simulink model "pendulumTest"  (R2021a)
settings: Solver=VariableStepAuto  StartTime=0.0  StopTime=10.0  FixedStep=1/20000  RelTol=1e-3
InitFcn:
  | run('init.m');
values from neighbouring files (symbols this model uses):
  g = 9.81    [init.m]
  l = 0.5    [init.m]
  m = 1    [init.m]
  Q = 1e-5    (= 1e-05)    [init.m]
  R = 1e-3    (= 0.001)    [init.m]
  Ts = 1/2000    (= 0.0005)    [init.m]
undefined symbols (not defined in the file or in its folder): A, B, Discrete, H, Time, X, Y, Z
libraries: sm_lib x8, nesl_utility x3, simulink x2, ctrlSharedLib x1
settings Model: Creator=Max  LastModifiedBy=Max

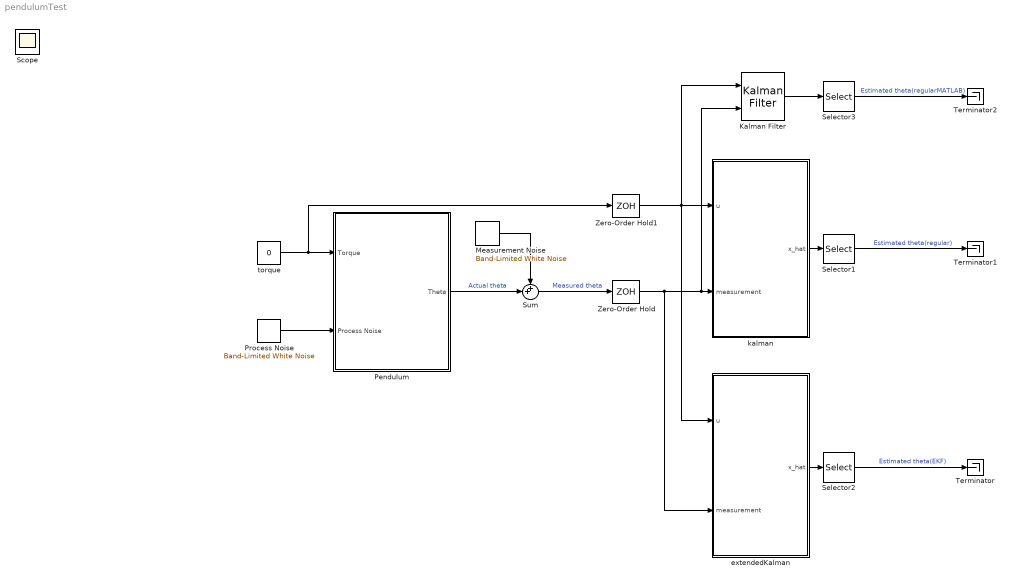
== system pendulumTest ==
  Kalman Filter : ctrlSharedLib/Kalman Filter  TimeDomain=Discrete-Time  UseCurrentEstimator=on  ModelSource=Individual A, B, C, D matrices  ModelSourceVariable=ss(0.95,1,1,0,1)  A=A  B=B  C=H  D=0  NumberOfStates=1  NumberOfInputs=1  NumberOfOutputs=1  InitialEstimateSource=Dialog  X0=0  P0=10  UseK=off  UseGH=off  NumberOfProcessNoiseInputs=1  G=1  TimeInvariantG=on  H=0  TimeInvariantH=on  Q=diag([0 Q])  TimeInvariantQ=on  R=R  TimeInvariantR=on  N=0  TimeInvariantN=on  AddInputPort=on  AddEnablePort=off  OutputEstimatedY=off  OutputP=off  Ts=Ts
  Measurement Noise : simulink/Sources/Band-Limited White Noise  Cov=R*Ts  Ts=Ts  seed=[12347]
  Pendulum : Subsystem  mask{theta_0=0.75*pi, theta_dot_0=0}
      mask prompts: theta_0 "Initial value of theta"; theta_dot_0 "Initial value of theta_dot"
      mask Display:
      | port_label('input',1,'T');
      | port_label('input',2,'w');
      | port_label('output',1,'\theta','interpreter','tex');
  Process Noise : simulink/Sources/Band-Limited White Noise  Cov=Q*Ts  Ts=Ts  seed=[23341]
  Selector1 : Selector  InputPortWidth=2  IndexOptions=Index vector (dialog)  Indices=1  OutputSizes=1
  Selector2 : Selector  InputPortWidth=2  IndexOptions=Index vector (dialog)  Indices=1  OutputSizes=1
  Selector3 : Selector  InputPortWidth=2  IndexOptions=Index vector (dialog)  Indices=1  OutputSizes=1
  Sum : Sum  Inputs=++|
  Terminator : Terminator
  Terminator1 : Terminator
  Terminator2 : Terminator
  Zero-Order Hold : ZeroOrderHold  SampleTime=Ts
  Zero-Order Hold1 : ZeroOrderHold  SampleTime=Ts
  extendedKalman : MATLAB Function  TreatAsAtomicUnit=on
  kalman : MATLAB Function  TreatAsAtomicUnit=on
  torque : Constant  Value=0
  Scope : Scope
  wires:
  kalman/1(x_hat) -> Selector1/1
  Pendulum/1(Theta) -> Sum/2  "Actual theta"
  Selector1/1 -> Terminator1/1  "Estimated theta(regular)"
  Sum/1 -> Zero-Order Hold/1  "Measured theta"
  Process Noise/1 -> Pendulum/2(Process Noise)
  Selector2/1 -> Terminator/1  "Estimated theta(EKF)"
  Measurement Noise/1 -> Sum/1
  torque/1 -> Pendulum/1(Torque), Zero-Order Hold1/1
  Zero-Order Hold/1 -> extendedKalman/2(measurement), Kalman Filter/2, kalman/2(measurement)
  Zero-Order Hold1/1 -> kalman/1(u), extendedKalman/1(u), Kalman Filter/1
  extendedKalman/1(x_hat) -> Selector2/1
  Kalman Filter/1 -> Selector3/1
  Selector3/1 -> Terminator2/1  "Estimated theta(regularMATLAB)"

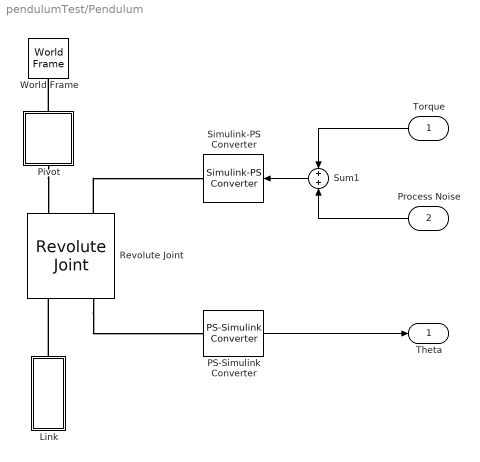
== system pendulumTest/Pendulum ==
  Torque : Inport
  Process Noise : Inport  Port=2
  Link : Subsystem  Tag=CustomStyle
  PS-Simulink Converter : nesl_utility/PS-Simulink Converter  PhysicalDomain=network_engine_domain  SubClassName=ps_output  LeftPortType=input  RightPortType=output  PseudoPeriodic=off  Frequencies=[]  Unit=1  AffineConversion=off
  Pivot : Subsystem  Tag=CustomStyle
  Revolute Joint : sm_lib/Joints/Revolute Joint  JointMode=Normal  SenseConstraintForce=off  SenseConstraintForceX=off  SenseConstraintForceY=off  SenseConstraintForceZ=off  SenseConstraintTorque=off  SenseConstraintTorqueX=off  SenseConstraintTorqueY=off  SenseConstraintTorqueZ=off  SenseTotalForce=off  SenseTotalForceX=off  SenseTotalForceY=off  SenseTotalForceZ=off  SenseTotalTorque=off  SenseTotalTorqueX=off  SenseTotalTorqueY=off  SenseTotalTorqueZ=off  CompositeWrenchDir=FollowerOnBase  CompositeWrenchFrame=BaseFrame  EquilibriumPosition=0  EquilibriumPositionUnits=rad  SpringStiffness=0  SpringStiffnessUnits=N*m/rad  DampingCoefficient=0  DampingCoefficientUnits=N*m/(rad/s)  TorqueActuationMode=InputTorque  MotionActuationMode=ComputedMotion  SensePosition=on  SenseVelocity=off  SenseAcceleration=off  SenseTorqueForce=off  SenseLowerLimitTorqueForce=off  SenseUpperLimitTorqueForce=off  LowerLimitSpecify=off  LowerLimitBound=-90  LowerLimitBoundUnits=deg  LowerLimitStiffness=1e4  LowerLimitStiffnessUnits=N*m/deg  LowerLimitDamping=10  LowerLimitDampingUnits=N*m/(deg/s)  LowerLimitTransitionRegionWidth=0.1  LowerLimitTransitionRegionWidthUnits=deg  UpperLimitSpecify=off  UpperLimitBound=90  UpperLimitBoundUnits=deg  UpperLimitStiffness=1e4  UpperLimitStiffnessUnits=N*m/deg  UpperLimitDamping=10  UpperLimitDampingUnits=N*m/(deg/s)  UpperLimitTransitionRegionWidth=0.1  UpperLimitTransitionRegionWidthUnits=deg  PositionTargetSpecify=on  PositionTargetPriority=High  PositionTargetValue=theta_0  PositionTargetValueUnits=rad  VelocityTargetSpecify=on  VelocityTargetPriority=High  VelocityTargetValue=theta_dot_0  VelocityTargetValueUnits=rad/s
  Simulink-PS Converter : nesl_utility/Simulink-PS Converter  PhysicalDomain=network_engine_domain  SubClassName=ps_input  LeftPortType=input  RightPortType=output  PseudoPeriodic=off  Frequencies=[]  NoiseDistribution=none  NoiseParameters=[]  Unit=1  AffineConversion=off  FilteringAndDerivatives=provide  SimscapeFilterOrder=1  InputFilterTimeConstant=0.001  UdotUserProvided=0
  Sum1 : Sum  Inputs=+|+
  World Frame : sm_lib/Frames and Transforms/World Frame
  Theta : Outport
  wires:
  Sum1/1 -> Simulink-PS Converter/1
  Torque/1 -> Sum1/1
  Process Noise/1 -> Sum1/2
  PS-Simulink Converter/1 -> Theta/1
  connections:
  Revolute Joint/LConn2 -- Simulink-PS Converter/RConn1
  Pivot/LConn1 -- World Frame/RConn1
  Pivot/RConn1 -- Revolute Joint/LConn1
  Link/RConn1 -- Revolute Joint/RConn1
  Revolute Joint/RConn2 -- PS-Simulink Converter/LConn1

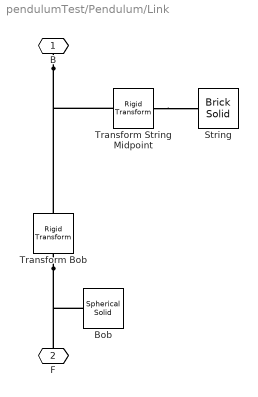
== system pendulumTest/Pendulum/Link ==
  Bob : sm_lib/Body Elements/Spherical Solid  GraphicAmbientColor=[0.15 0.15 0.15 1.0]  BasedOnType=Density  CenterOfMass=[0 0 0]  CenterOfMassUnits=m  GraphicDiffuseColor=[1.0 0.2 0.0]  Density=1000  DensityUnits=kg/(m^3)  DoExposeReferenceFrame=on  GraphicEmissiveColor=[0.0 0.0 0.0 1.0]  ExportEntireGeometry=off  SerializedExposedGeometries=<ExposedGeometries/>  SerializedFrames=<Frames/>  MarkerShape=Sphere  MarkerSize=10  GraphicType=FromGeometry  InertiaType=PointMass  Mass=m  MassUnits=kg  MomentsOfInertia=[1 1 1]*1e-3  MomentsOfInertiaUnits=kg*m^2  GraphicOpacity=1.0  ProductsOfInertia=[0 0 0]  ProductsOfInertiaUnits=kg*m^2  GraphicShininess=75  GraphicSpecularColor=[0.5 0.5 0.5 1.0]  SphereRadius=0.05  SphereRadiusUnits=m  GraphicVisPropType=SimpleVisualProperties
  String : sm_lib/Body Elements/Brick Solid  GraphicAmbientColor=[0.15 0.15 0.15 1.0]  BasedOnType=Density  BrickDimensions=[0.01 l 0.01]  BrickDimensionUnits=m  CenterOfMass=[0 0 0]  CenterOfMassUnits=m  GraphicDiffuseColor=[1.0 0.2 0.0]  Density=0  DensityUnits=kg/(m^3)  DoExposeReferenceFrame=on  GraphicEmissiveColor=[0.0 0.0 0.0 1.0]  ExportEntireGeometry=off  SerializedFrames=<Frames/>  MarkerShape=Sphere  MarkerSize=10  GraphicType=FromGeometry  InertiaType=CalculateFromGeometry  Mass=0  MassUnits=kg  MomentsOfInertia=[1 1 1]*1e-3  MomentsOfInertiaUnits=kg*m^2  GraphicOpacity=1.0  ProductsOfInertia=[0 0 0]  ProductsOfInertiaUnits=kg*m^2  GraphicShininess=75  GraphicSpecularColor=[0.5 0.5 0.5 1.0]  GraphicVisPropType=SimpleVisualProperties
  "Transform Bob " : sm_lib/Frames and Transforms/Rigid Transform  TranslationMethod=StandardAxis  TranslationStandardOffset=l  TranslationLengthUnit=m  TranslationStandardAxis=-Y  TranslationCartesianOffset=[0 0 0]  TranslationROffset=0  TranslationROffsetUnits=m  TranslationZOffset=0  TranslationZOffsetUnits=m  TranslationThetaOffset=0  TranslationThetaOffsetUnits=deg  RotationMethod=None  RotationAngleUnits=deg  RotationStandardAxis=+Z  RotationAngle=0  RotationArbitraryAxis=[0 0 1]  FollAlignAxisA=+X  BaseAlignAxisA=+Y  FollAlignAxisB=+Y  BaseAlignAxisB=+Z  RotationSequenceAxes=FollowerAxes  RotationSequence=XYX  RotationSequenceAngles=[0 0 0]  RotationSequenceAnglesUnits=deg  RotationMatrix=[1 0 0; 0 1 0; 0 0 1]
  Transform String Midpoint : sm_lib/Frames and Transforms/Rigid Transform  TranslationMethod=StandardAxis  TranslationStandardOffset=l/2  TranslationLengthUnit=m  TranslationStandardAxis=-Y  TranslationCartesianOffset=[0 0 0]  TranslationROffset=0  TranslationROffsetUnits=m  TranslationZOffset=0  TranslationZOffsetUnits=m  TranslationThetaOffset=0  TranslationThetaOffsetUnits=deg  RotationMethod=None  RotationAngleUnits=deg  RotationStandardAxis=+Z  RotationAngle=0  RotationArbitraryAxis=[0 0 1]  FollAlignAxisA=+X  BaseAlignAxisA=+Y  FollAlignAxisB=+Y  BaseAlignAxisB=+Z  RotationSequenceAxes=FollowerAxes  RotationSequence=XYX  RotationSequenceAngles=[0 0 0]  RotationSequenceAnglesUnits=deg  RotationMatrix=[1 0 0; 0 1 0; 0 0 1]
  B : PMIOPort  Side=Right
  F : PMIOPort  Port=2  Side=Left
  connections:
  Transform String Midpoint/RConn1 -- String/RConn1
  "Transform Bob "/RConn1 -- F/RConn1 -- Bob/RConn1
  B/RConn1 -- Transform String Midpoint/LConn1 -- "Transform Bob "/LConn1

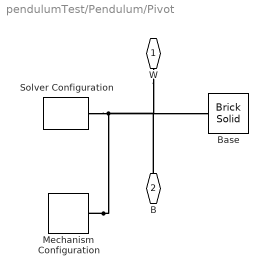
== system pendulumTest/Pendulum/Pivot ==
  Base : sm_lib/Body Elements/Brick Solid  GraphicAmbientColor=[0.15 0.15 0.15 1.0]  BasedOnType=Density  BrickDimensions=[0.2 0.05 0.1]  BrickDimensionUnits=m  CenterOfMass=[0 0 0]  CenterOfMassUnits=m  GraphicDiffuseColor=[0.2 0.2 0.2]  Density=1000  DensityUnits=kg/(m^3)  DoExposeReferenceFrame=on  GraphicEmissiveColor=[0.0 0.0 0.0 1.0]  ExportEntireGeometry=off  SerializedFrames=<Frames/>  MarkerShape=Sphere  MarkerSize=10  GraphicType=FromGeometry  InertiaType=CalculateFromGeometry  Mass=1  MassUnits=kg  MomentsOfInertia=[1 1 1]*1e-3  MomentsOfInertiaUnits=kg*m^2  GraphicOpacity=1.0  ProductsOfInertia=[0 0 0]  ProductsOfInertiaUnits=kg*m^2  GraphicShininess=75  GraphicSpecularColor=[0.5 0.5 0.5 1.0]  GraphicVisPropType=SimpleVisualProperties
  Mechanism Configuration : sm_lib/Utilities/Mechanism Configuration  UniformGravity=Constant  GravityVector=[0 -g 0]  GravityVectorUnits=m/s^2  GravityUnits=m/s^2  LinearizationDelta=0.001  JointModeTransitionNonlinearIterations=2
  Solver Configuration : nesl_utility/Solver Configuration  PhysicalDomain=network_engine_domain  SubClassName=solver  LeftPortType=input  RightPortType=generic  Tones=[]  Harmonics=[]  SimulateNoise=off  Profile=off  UseLocalSampling=off  EnableSwitchedLinearOptims=on  FrequencyDomain=off  UseCCode=off  RelTol=0.001  AbsTol=1e-06  MinStep=1e-09  ToWorkspace=off  RevertToSquareIcSolve=off  NumHomotopyIterations=100  PhasorMode=off  PhasorModeNumHarmonics=1  DoDC=off  ResidualTolerance=1e-9  UseLocalSolver=off  LocalSolverChoice=NE_BACKWARD_EULER_ADVANCER  LocalSolverSampleTime=.001  DoFixedCost=off  MaxNonlinIter=3  MaxModeIter=2  ComputeImpulses=off  ImpulseIterations=2  LinearAlgebra=Sparse  EquationFormulation=NE_TIME_EF  DelaysMemoryBudget=1024  AutomaticFiltering=on  FilteringTimeConstant=0.001  PartitionStorageMethod=AS_NEEDED  PartitionMemoryBudget=1024  PartitionMethod=FAST
  W : PMIOPort  Side=Left
  B : PMIOPort  Port=2  Side=Right
  connections:
  Mechanism Configuration/RConn1 -- Solver Configuration/RConn1 -- B/RConn1 -- Base/RConn1 -- W/RConn1

== matlab function pendulumTest/extendedKalman ==
  data: u input; x_hat output; measurement input
function x_hat = extendedKalman_function(u, measurement)
    persistent x_hat_prev P_prev
    
    if isempty(x_hat_prev)
        x_hat_prev = [0; 0];
        P_prev = eye(2)*1e-3;
    end
    
    % Pendulum model
    A = [0 1; -(9.81/0.5)*sin(x_hat_prev(1)) 0];
    B = [0; 1/(1*0.5^2)];
    H = [1 0];
    D = 0;
    % Process noise covariance
    Q = diag([0 1e-3]);
    % Measurement noise covariance
    R = 1e-4;
    
    % Make the model discrete
    Ts = 1/2000; % sec
    A = eye(2)+Ts*A;
    F = eye(2)+Ts*[0 1; -(9.81/0.5)*cos(x_hat_prev(1)) 0];
    B = Ts*B;
    
    % Prediction step
    x_minus = A * x_hat_prev + B * u;
    P_minus = F * P_prev * F' + Q;

    % Update step
    K = P_minus * H' / (H * P_minus * H' + R);
    x_hat = x_minus + K * (measurement - H * x_minus);
    P = (eye(2) - K * H) * P_minus;

    % Update persistent variables for the next iteration
    x_hat_prev = x_hat;
    P_prev = P;
end

== matlab function pendulumTest/kalman ==
  data: u input; x_hat output; measurement input
function x_hat = kalman_function(u, measurement)
    persistent x_hat_prev P_prev
    
    if isempty(x_hat_prev)
        x_hat_prev = [0; 0];
        P_prev = eye(2)*1e-3;
    end
    
    % Pendulum model
    A = [0 1; -(9.81/0.5) 0];
    B = [0; 1/(1*0.5^2)];
    H = [1 0];
    D = 0;
    % Process noise covariance
    Q = diag([0 1e-3]);
    % Measurement noise covariance
    R = 1e-4;
    
    % Make the model discrete
    Ts = 1/2000; % sec
    A = eye(2)+Ts*A;
    F = A;
    B = Ts*B;
    
    % Prediction step
    x_minus = A * x_hat_prev + B * u;
    P_minus = F * P_prev * F' + Q;

    % Update step
    K = P_minus * H' / (H * P_minus * H' + R);
    x_hat = x_minus + K * (measurement - H * x_minus);
    P = (eye(2) - K * H) * P_minus;

    % Update persistent variables for the next iteration
    x_hat_prev = x_hat;
    P_prev = P;
end
